simulink model "nonlin_unique_plane"  (Simulink 6.0)
settings: Solver=ode45  StartTime=0.0  StopTime=300  RelTol=1e-3
undefined symbols (not defined in the file): B, DQ, DQL, I, m, M, Ma, MaU, rg, T, W, xb, xg, Xudot, yb, yg, Yvdot, zb, zg, Zwdot
libraries: simulink x24, rov_design_analysis x16
(part 1 of 3)
settings Model: LastModifiedBy=c chin

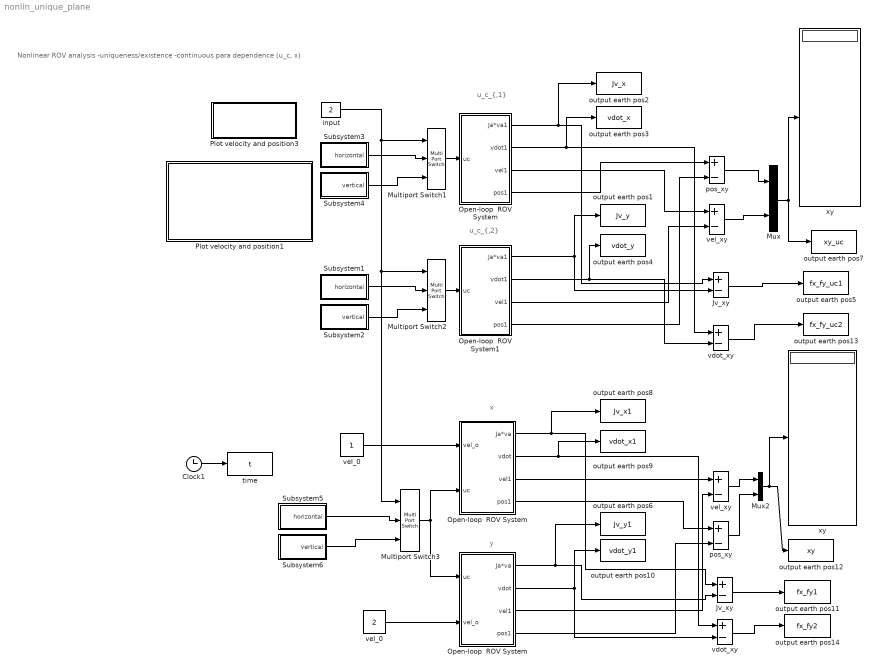
== system nonlin_unique_plane ==
  note: Nonlinear ROV analysis
      | -uniqueness/existence
      | -continuous para dependence (u_c, x)
  note: u_c_{,1}
  note: x
  note: y
  note: u_c_{,2}
  Clock1 : Clock
      settings: Decimation=10
  Jv_xy : Sum  Inputs=+-  SaturateOnIntegerOverflow=on  InputSameDT=on
  "Jv_xy " : Sum  Inputs=+-  SaturateOnIntegerOverflow=on  InputSameDT=on
  Multiport Switch1 : MultiPortSwitch  Inputs=2
  Multiport Switch2 : MultiPortSwitch  Inputs=2
  Multiport Switch3 : MultiPortSwitch  Inputs=2
  Mux : Mux  Inputs=2
  Mux2 : Mux  Inputs=2
  Open-loop  ROV System : Subsystem
  "Open-loop  ROV System   " : Subsystem
  "Open-loop  ROV System     " : Subsystem
  Open-loop  ROV System1 : Subsystem
  Plot velocity and position1 : Subsystem
      settings: OpenFcn=|
      | clc
      | cd C:\Matlab7\toolbox\rov_design_analysis\nonlin_analysis
      | run unique_analy_plane
      mask Display: disp('Double-click \n to \n check \n 1. uniqueness/existence \n 2. continuous  para. dependence\n HORT/VERT')
  Plot velocity and position3 : Subsystem  AncestorBlock=|
      | rov_design_analysis/ROV Controller
      | Design
      | Applications/Plot velocity and position
      settings: OpenFcn=|
      | clc
      | cd c:\Matlab7\toolbox\rov_design_analysis\hybrid
      | sim('nonlin_unique_plane')
      mask Display: disp('Run  SIMULINK')
  Subsystem1 : Subsystem
  Subsystem2 : Subsystem
  Subsystem3 : Subsystem
  Subsystem4 : Subsystem
  Subsystem5 : Subsystem
  Subsystem6 : Subsystem
  "input " : Constant  Value=2
  output earth pos1 : ToWorkspace  VariableName=Jv_y  SampleTime=1  SaveFormat=Array
  output earth pos10 : ToWorkspace  VariableName=vdot_y1  SampleTime=1  SaveFormat=Array
  output earth pos11 : ToWorkspace  VariableName=fx_fy1  SampleTime=1  SaveFormat=Array
  output earth pos12 : ToWorkspace  VariableName=xy  SampleTime=1  SaveFormat=Array
  output earth pos13 : ToWorkspace  VariableName=fx_fy_uc2  SampleTime=1  SaveFormat=Array
  output earth pos14 : ToWorkspace  VariableName=fx_fy2  SampleTime=1  SaveFormat=Array
  output earth pos2 : ToWorkspace  VariableName=Jv_x  SampleTime=1  SaveFormat=Array
  output earth pos3 : ToWorkspace  VariableName=vdot_x  SampleTime=1  SaveFormat=Array
  output earth pos4 : ToWorkspace  VariableName=vdot_y  SampleTime=1  SaveFormat=Array
  output earth pos5 : ToWorkspace  VariableName=fx_fy_uc1  SampleTime=1  SaveFormat=Array
  output earth pos6 : ToWorkspace  VariableName=Jv_y1  SampleTime=1  SaveFormat=Array
  output earth pos7 : ToWorkspace  VariableName=xy_uc  SampleTime=1  SaveFormat=Array
  output earth pos8 : ToWorkspace  VariableName=Jv_x1  SampleTime=1  SaveFormat=Array
  output earth pos9 : ToWorkspace  VariableName=vdot_x1  SampleTime=1  SaveFormat=Array
  pos_xy : Sum  Inputs=+-  SaturateOnIntegerOverflow=on  InputSameDT=on
  "pos_xy " : Sum  Inputs=+-  SaturateOnIntegerOverflow=on  InputSameDT=on
  time : ToWorkspace  VariableName=t  SampleTime=1  SaveFormat=Array
  vdot_xy : Sum  Inputs=+-  SaturateOnIntegerOverflow=on  InputSameDT=on
  "vdot_xy " : Sum  Inputs=+-  SaturateOnIntegerOverflow=on  InputSameDT=on
  vel_0 : Constant  Value=2
  "vel_0 " : Constant
  vel_xy : Sum  Inputs=+-  SaturateOnIntegerOverflow=on  InputSameDT=on
  "vel_xy " : Sum  Inputs=+-  SaturateOnIntegerOverflow=on  InputSameDT=on
  xy : Display
  "xy  " : Display
  wires:
  Clock1/1 -> time/1
  "vel_xy "/1 -> Mux2/1
  "pos_xy "/1 -> Mux2/2
  Mux2/1 -> output earth pos12/1, "xy  "/1
  "vel_0 "/1 -> "Open-loop  ROV System   "/1(vel_o)
  vel_0/1 -> "Open-loop  ROV System     "/2(vel_o)
  Multiport Switch1/1 -> Open-loop  ROV System/1(uc)
  Open-loop  ROV System/1(Ja*va1) -> Jv_xy/1, output earth pos2/1
  Open-loop  ROV System1/1(Ja*va1) -> Jv_xy/2, output earth pos1/1
  Open-loop  ROV System/2(vdot1) -> vdot_xy/1, output earth pos3/1
  Open-loop  ROV System1/2(vdot1) -> vdot_xy/2, output earth pos4/1
  Open-loop  ROV System/4("pos1 ") -> pos_xy/1
  Open-loop  ROV System1/4("pos1 ") -> pos_xy/2
  Open-loop  ROV System/3("vel1 ") -> vel_xy/1
  Open-loop  ROV System1/3("vel1 ") -> vel_xy/2
  pos_xy/1 -> Mux/1
  vel_xy/1 -> Mux/2
  "Open-loop  ROV System   "/1(Ja*va) -> "Jv_xy "/1, output earth pos8/1
  "Open-loop  ROV System     "/1(Ja*va) -> "Jv_xy "/2, output earth pos6/1
  "Open-loop  ROV System   "/3(vel1) -> "vel_xy "/1
  "Open-loop  ROV System     "/3(vel1) -> "vel_xy "/2
  "Open-loop  ROV System   "/4(pos1) -> "pos_xy "/1
  "Open-loop  ROV System     "/4(pos1) -> "pos_xy "/2
  Jv_xy/1 -> output earth pos5/1
  vdot_xy/1 -> output earth pos13/1
  "Jv_xy "/1 -> output earth pos11/1
  "vdot_xy "/1 -> output earth pos14/1
  "Open-loop  ROV System   "/2(vdot) -> "vdot_xy "/1, output earth pos9/1
  "Open-loop  ROV System     "/2(vdot) -> "vdot_xy "/2, output earth pos10/1
  Mux/1 -> output earth pos7/1, xy/1
  Multiport Switch2/1 -> Open-loop  ROV System1/1(uc)
  Multiport Switch3/1 -> "Open-loop  ROV System   "/2(uc), "Open-loop  ROV System     "/1(uc)
  Subsystem4/1(vertical) -> Multiport Switch1/3
  Subsystem3/1(horizontal) -> Multiport Switch1/2
  "input "/1 -> Multiport Switch1/1, Multiport Switch2/1, Multiport Switch3/1
  Subsystem2/1(vertical) -> Multiport Switch2/3
  Subsystem1/1(horizontal) -> Multiport Switch2/2
  Subsystem6/1(vertical) -> Multiport Switch3/3
  Subsystem5/1(horizontal) -> Multiport Switch3/2

== system nonlin_unique_plane/Open-loop  ROV System ==
  uc : Inport  Port=1  LatchInput=off
  " Six DOF RRC ROV   " : Subsystem
      mask Display:
      | disp('ROV')
      | image(imread('/rov_design_analysis/fig/ROVRRC2.jpg'));
      | color('white');port_label('input',2,'thrust')
      | color('white');port_label('input',1,'MCD_select')
      | color('white');port_label('input',3,'pos')
      | color('white');port_label('output',1,'vel')
      | color('white');port_label('output',2,'vel_dot')
  Body Velocity Scope  1 : Subsystem  AncestorBlock=|
      | rov_design_analysis/Scope
      | Utilities/Body Velocity
      | Scope
      mask Display: disp('Body\nVelocity\nScope')
  "Euler Transformation  " : Subsystem  AncestorBlock=rov_design_analysis/Scope Utilities/Euler Transformation
  Thruster configuration5 : Subsystem
      mask Display: disp('T')
  Thruster configuration8 : Subsystem  AncestorBlock=|
      | rov_design_analysis/ROV Controller
      | Design
      | Applications/1. Heading autopilot/Thruster
      | configuration
      mask Display: disp('F_T')
  "input " : Constant  Value=2
  Ja*va1 : Outport
  vdot1 : Outport  Port=2
  "vel1 " : Outport  Port=3
  "pos1 " : Outport  Port=4
  wires:
  "Euler Transformation  "/1(eout) -> Body Velocity Scope  1/1(In), "pos1 "/1, " Six DOF RRC ROV   "/3("pos ")
  " Six DOF RRC ROV   "/1(vel) -> "Euler Transformation  "/1(vel), "vel1 "/1
  " Six DOF RRC ROV   "/2(vel_dot) -> vdot1/1
  "Euler Transformation  "/2(eout_dot) -> Ja*va1/1
  Thruster configuration8/1(output force) -> Thruster configuration5/1(input velocity)
  Thruster configuration5/1(output force) -> " Six DOF RRC ROV   "/2("thrust ")
  uc/1 -> Thruster configuration8/1(input velocity)
  "input "/1 -> " Six DOF RRC ROV   "/1(MCD_select)

== system nonlin_unique_plane/Open-loop  ROV System    ==
  vel_o : Inport  Port=1  LatchInput=off
  uc : Inport  Port=2  LatchInput=off
  " Six DOF RRC ROV   " : Subsystem
      mask Display:
      | disp('ROV')
      | image(imread('/rov_design_analysis/fig/ROVRRC2.jpg'));
      | color('white');port_label('input',2,'thrust')
      | color('white');port_label('input',1,'MCD_select')
      | color('white');port_label('input',3,'pos')
      | color('white');port_label('output',1,'vel')
      | color('white');port_label('output',2,'vel_dot')
  Body Velocity Scope  1 : Subsystem  AncestorBlock=|
      | rov_design_analysis/Scope
      | Utilities/Body Velocity
      | Scope
      mask Display: disp('Body\nVelocity\nScope')
  "Euler Transformation  " : Subsystem  AncestorBlock=rov_design_analysis/Scope Utilities/Euler Transformation
  Thruster configuration5 : Subsystem
      mask Display: disp('T')
  Thruster configuration8 : Subsystem  AncestorBlock=|
      | rov_design_analysis/ROV Controller
      | Design
      | Applications/1. Heading autopilot/Thruster
      | configuration
      mask Display: disp('F_T')
  "input " : Constant  Value=2
  Ja*va : Outport
  vdot : Outport  Port=2
  vel1 : Outport  Port=3
  pos1 : Outport  Port=4
  wires:
  "Euler Transformation  "/1(eout) -> pos1/1, " Six DOF RRC ROV   "/3("pos "), Body Velocity Scope  1/1(In)
  " Six DOF RRC ROV   "/1(vel) -> "Euler Transformation  "/1(vel), vel1/1
  "Euler Transformation  "/2(Ja*va) -> Ja*va/1
  " Six DOF RRC ROV   "/2(vel_dot) -> vdot/1
  vel_o/1 -> " Six DOF RRC ROV   "/4(v0)
  Thruster configuration8/1(output force) -> Thruster configuration5/1(input velocity)
  Thruster configuration5/1(output force) -> " Six DOF RRC ROV   "/2("thrust ")
  uc/1 -> Thruster configuration8/1(input velocity)
  "input "/1 -> " Six DOF RRC ROV   "/1(MCD_select)

== system nonlin_unique_plane/Open-loop  ROV System      ==
  uc : Inport  Port=1  LatchInput=off
  vel_o : Inport  Port=2  LatchInput=off
  " Six DOF RRC ROV   " : Subsystem
      mask Display:
      | disp('ROV')
      | image(imread('/rov_design_analysis/fig/ROVRRC2.jpg'));
      | color('white');port_label('input',2,'thrust')
      | color('white');port_label('input',1,'MCD_select')
      | color('white');port_label('input',3,'pos')
      | color('white');port_label('output',1,'vel')
      | color('white');port_label('output',2,'vel_dot')
  Body Velocity Scope  1 : Subsystem  AncestorBlock=|
      | rov_design_analysis/Scope
      | Utilities/Body Velocity
      | Scope
      mask Display: disp('Body\nVelocity\nScope')
  "Euler Transformation  " : Subsystem  AncestorBlock=rov_design_analysis/Scope Utilities/Euler Transformation
  Thruster configuration5 : Subsystem
      mask Display: disp('T')
  Thruster configuration8 : Subsystem  AncestorBlock=|
      | rov_design_analysis/ROV Controller
      | Design
      | Applications/1. Heading autopilot/Thruster
      | configuration
      mask Display: disp('F_T')
  "input " : Constant  Value=2
  Ja*va : Outport
  vdot : Outport  Port=2
  vel1 : Outport  Port=3
  pos1 : Outport  Port=4
  wires:
  "Euler Transformation  "/1(eout) -> pos1/1, " Six DOF RRC ROV   "/3("pos "), Body Velocity Scope  1/1(In)
  " Six DOF RRC ROV   "/1(vel) -> "Euler Transformation  "/1(vel), vel1/1
  "Euler Transformation  "/2(Ja*va) -> Ja*va/1
  " Six DOF RRC ROV   "/2(vel_dot) -> vdot/1
  vel_o/1 -> " Six DOF RRC ROV   "/4(v0)
  Thruster configuration8/1(output force) -> Thruster configuration5/1(input velocity)
  Thruster configuration5/1(output force) -> " Six DOF RRC ROV   "/2("thrust ")
  uc/1 -> Thruster configuration8/1(input velocity)
  "input "/1 -> " Six DOF RRC ROV   "/1(MCD_select)

== system nonlin_unique_plane/Open-loop  ROV System1 ==
  uc : Inport  Port=1  LatchInput=off
  " Six DOF RRC ROV   " : Subsystem
      mask Display:
      | disp('ROV')
      | image(imread('/rov_design_analysis/fig/ROVRRC2.jpg'));
      | color('white');port_label('input',2,'thrust')
      | color('white');port_label('input',1,'MCD_select')
      | color('white');port_label('input',3,'pos')
      | color('white');port_label('output',1,'vel')
      | color('white');port_label('output',2,'vel_dot')
  Body Velocity Scope  1 : Subsystem  AncestorBlock=|
      | rov_design_analysis/Scope
      | Utilities/Body Velocity
      | Scope
      mask Display: disp('Body\nVelocity\nScope')
  "Euler Transformation  " : Subsystem  AncestorBlock=rov_design_analysis/Scope Utilities/Euler Transformation
  Thruster configuration5 : Subsystem
      mask Display: disp('T')
  Thruster configuration8 : Subsystem  AncestorBlock=|
      | rov_design_analysis/ROV Controller
      | Design
      | Applications/1. Heading autopilot/Thruster
      | configuration
      mask Display: disp('F_T')
  "input " : Constant  Value=2
  Ja*va1 : Outport
  vdot1 : Outport  Port=2
  "vel1 " : Outport  Port=3
  "pos1 " : Outport  Port=4
  wires:
  "Euler Transformation  "/1(eout) -> "pos1 "/1, Body Velocity Scope  1/1(In), " Six DOF RRC ROV   "/3("pos ")
  " Six DOF RRC ROV   "/1(vel) -> "Euler Transformation  "/1(vel), "vel1 "/1
  " Six DOF RRC ROV   "/2(vel_dot) -> vdot1/1
  "Euler Transformation  "/2(eout_dot) -> Ja*va1/1
  Thruster configuration8/1(output force) -> Thruster configuration5/1(input velocity)
  Thruster configuration5/1(output force) -> " Six DOF RRC ROV   "/2("thrust ")
  uc/1 -> Thruster configuration8/1(input velocity)
  "input "/1 -> " Six DOF RRC ROV   "/1(MCD_select)

== system nonlin_unique_plane/Plot velocity and position1 ==

== system nonlin_unique_plane/Plot velocity and position3 ==

== system nonlin_unique_plane/Subsystem1 ==
  Mux1 : Mux
  u1 : Step  Time=0  After=2  SampleTime=0
  u2 : Step  Time=0  After=2  SampleTime=0
  u3 : Step  Time=0  After=0  SampleTime=0
  u4 : Step  Time=0  After=0  SampleTime=0
  horizontal : Outport
  wires:
  u2/1 -> Mux1/2
  u1/1 -> Mux1/1
  u3/1 -> Mux1/3
  Mux1/1 -> horizontal/1
  u4/1 -> Mux1/4

== system nonlin_unique_plane/Subsystem2 ==
  Mux1 : Mux
  u1 : Step  Time=0  After=0  SampleTime=0
  u2 : Step  Time=0  After=0  SampleTime=0
  u3 : Step  Time=0  After=2  SampleTime=0
  u4 : Step  Time=0  After=2  SampleTime=0
  vertical : Outport
  wires:
  u2/1 -> Mux1/2
  u1/1 -> Mux1/1
  u3/1 -> Mux1/3
  u4/1 -> Mux1/4
  Mux1/1 -> vertical/1

== system nonlin_unique_plane/Subsystem3 ==
  Mux1 : Mux
  u1 : Step  Time=0  SampleTime=0
  u2 : Step  Time=0  SampleTime=0
  u3 : Step  Time=0  After=0  SampleTime=0
  u4 : Step  Time=0  After=0  SampleTime=0
  horizontal : Outport
  wires:
  u2/1 -> Mux1/2
  u1/1 -> Mux1/1
  u3/1 -> Mux1/3
  Mux1/1 -> horizontal/1
  u4/1 -> Mux1/4

== system nonlin_unique_plane/Subsystem4 ==
  Mux1 : Mux
  u1 : Step  Time=0  After=0  SampleTime=0
  u2 : Step  Time=0  After=0  SampleTime=0
  u3 : Step  Time=0  SampleTime=0
  u4 : Step  Time=0  SampleTime=0
  vertical : Outport
  wires:
  u2/1 -> Mux1/2
  u1/1 -> Mux1/1
  u3/1 -> Mux1/3
  u4/1 -> Mux1/4
  Mux1/1 -> vertical/1

== system nonlin_unique_plane/Subsystem5 ==
  Mux1 : Mux
  u1 : Step  Time=0  SampleTime=0
  u2 : Step  Time=0  SampleTime=0
  u3 : Step  Time=0  After=0  SampleTime=0
  u4 : Step  Time=0  After=0  SampleTime=0
  horizontal : Outport
  wires:
  u2/1 -> Mux1/2
  u1/1 -> Mux1/1
  u3/1 -> Mux1/3
  Mux1/1 -> horizontal/1
  u4/1 -> Mux1/4

== system nonlin_unique_plane/Subsystem6 ==
  Mux1 : Mux
  u1 : Step  Time=0  After=0  SampleTime=0
  u2 : Step  Time=0  After=0  SampleTime=0
  u3 : Step  Time=0  SampleTime=0
  u4 : Step  Time=0  SampleTime=0
  vertical : Outport
  wires:
  u2/1 -> Mux1/2
  u1/1 -> Mux1/1
  u3/1 -> Mux1/3
  u4/1 -> Mux1/4
  Mux1/1 -> vertical/1

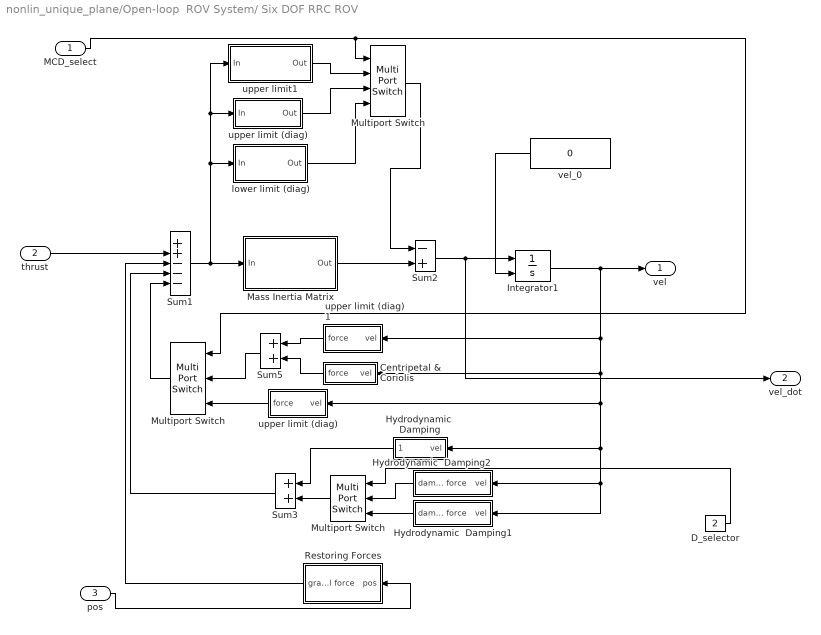
== system nonlin_unique_plane/Open-loop  ROV System/ Six DOF RRC ROV    ==
  MCD_select : Inport  Port=1  LatchInput=off
  "thrust " : Inport  Port=2  LatchInput=off
  "pos " : Inport  Port=3  LatchInput=off
  Centripetal & Coriolis : Subsystem  Orientation=left  AncestorBlock=rov_design_analysis/ROV Models/1. Six DOF RRC ROV II/Centripetal & Coriolis
      mask Display: disp('C')
  D_selector : Constant  Value=2
  Hydrodynamic  Damping : Subsystem  Orientation=left
      mask Display: disp('D')
  Hydrodynamic  Damping1 : Subsystem  Orientation=left
      mask Display: disp('perturb \nDamping')
  Hydrodynamic  Damping2 : Subsystem  Orientation=left
      mask Display: disp('Zero Perturb')
  Integrator1 : Integrator  InitialConditionSource=external
  Mass Inertia Matrix : Subsystem
      mask Display: disp('inv(MRB+MA)')
  Multiport Switch : MultiPortSwitch  Inputs=3
  "Multiport Switch  " : MultiPortSwitch  Orientation=left  Inputs=2
  "Multiport Switch    " : MultiPortSwitch  Orientation=left  Inputs=2
  Restoring Forces : Subsystem  Orientation=left
      mask Display: disp('Restoring\nForce')
  Sum1 : Sum  Inputs=++---  SaturateOnIntegerOverflow=on  InputSameDT=on
  Sum2 : Sum  Inputs=-+  SaturateOnIntegerOverflow=on  InputSameDT=on
  Sum3 : Sum  Orientation=left  SaturateOnIntegerOverflow=on  InputSameDT=on
  Sum5 : Sum  Orientation=left  SaturateOnIntegerOverflow=on  InputSameDT=on
  lower limit (diag) : Subsystem
      mask Display: disp('Perturb MA')
  upper limit (diag) : Subsystem
      mask Display: disp('Perturb MA')
  "upper limit (diag)   " : Subsystem  Orientation=left
      mask Display: disp('Perturb CA')
  upper limit (diag)   1 : Subsystem  Orientation=left
      mask Display: disp('CA')
  upper limit1 : Subsystem
      mask Display: disp('Zero Perturb')
  vel_0 : Constant  Orientation=left  Value=0  OutDataTypeMode=double
  vel : Outport
  vel_dot : Outport  Port=2
  wires:
  Restoring Forces/1(gravitational force) -> Sum1/3
  "thrust "/1 -> Sum1/2
  Sum1/1 -> Mass Inertia Matrix/1(In), upper limit1/1(In), upper limit (diag)/1(In), lower limit (diag)/1(In)
  "Multiport Switch  "/1 -> Sum1/5
  "pos "/1 -> Restoring Forces/1(pos)
  Mass Inertia Matrix/1(Out) -> Sum2/2
  upper limit1/1(Out) -> Multiport Switch/2
  upper limit (diag)/1(Out) -> Multiport Switch/3
  lower limit (diag)/1(Out) -> Multiport Switch/4
  Multiport Switch/1 -> Sum2/1
  "upper limit (diag)   "/1(force) -> "Multiport Switch  "/3
  Sum5/1 -> "Multiport Switch  "/2
  Hydrodynamic  Damping1/1(damping force) -> "Multiport Switch    "/3
  Hydrodynamic  Damping2/1(damping force) -> "Multiport Switch    "/2
  Sum3/1 -> Sum1/4
  "Multiport Switch    "/1 -> Sum3/2
  Hydrodynamic  Damping/1(damping force) -> Sum3/1
  MCD_select/1 -> Multiport Switch/1, "Multiport Switch  "/1
  upper limit (diag)   1/1(force) -> Sum5/1
  Centripetal & Coriolis/1(force) -> Sum5/2
  Sum2/1 -> Integrator1/1, vel_dot/1
  Integrator1/1 -> vel/1, upper limit (diag)   1/1(vel), Centripetal & Coriolis/1(vel), Hydrodynamic  Damping/1(vel), Hydrodynamic  Damping1/1(vel), Hydrodynamic  Damping2/1(vel), "upper limit (diag)   "/1(vel)
  vel_0/1 -> Integrator1/2
  D_selector/1 -> "Multiport Switch    "/1

== system nonlin_unique_plane/Open-loop  ROV System/Body Velocity Scope  1 ==
  In : Inport  Port=1  LatchInput=off
  Demux : Demux  Outputs=6
  p : Scope
      settings: TickLabels=on  YMin=-0.125  YMax=0.2  DataFormat=Array
  q : Scope
      settings: TickLabels=on  TimeRange=200  YMin=-0.05  YMax=0.15  DataFormat=Array
  r : Scope
      settings: TickLabels=on  TimeRange=200  YMin=-0.05  YMax=0.15  DataFormat=Array
  u : Scope
      settings: TickLabels=on  TimeRange=50  YMin=-0.025  YMax=0.375  DataFormat=Array
  v : Scope
      settings: TickLabels=on  YMin=-0.02  YMax=0.1  DataFormat=Array
  w : Scope
      settings: TickLabels=on  TimeRange=50  YMin=-0.0025  YMax=0.0375  DataFormat=Array
  wires:
  Demux/1 -> u/1
  Demux/2 -> v/1
  Demux/4 -> p/1
  Demux/3 -> w/1
  In/1 -> Demux/1
  Demux/5 -> q/1
  Demux/6 -> r/1

== system nonlin_unique_plane/Open-loop  ROV System/Euler Transformation   ==
  vel : Inport  Port=1  LatchInput=off
  Demux : Demux  Outputs=2
  Demux1 : Demux  Outputs=2
  Intregrator2 : Integrator
  Mux1 : Mux  Inputs=2
  Terminator : Terminator
  Transformation matrix R : Subsystem
      mask Display: disp('Transformation R')
  Transformation matrix T : Subsystem
      mask Display: disp('Transformation T')
  eout : Outport  InitialOutput=0
  eout_dot : Outport  Port=2  InitialOutput=0
  wires:
  Mux1/1 -> eout_dot/1, Intregrator2/1
  Intregrator2/1 -> Demux1/1, eout/1
  Demux/2 -> Transformation matrix R/1(angular body  velocity)
  Demux/1 -> Transformation matrix T/1(translational body velocity)
  vel/1 -> Demux/1
  Demux1/2 -> Transformation matrix T/2(angular position), Transformation matrix R/2(angular position)
  Transformation matrix R/1(angular earth velocity) -> Mux1/2
  Transformation matrix T/1(translational earth velocity) -> Mux1/1
  Demux1/1 -> Terminator/1

== system nonlin_unique_plane/Open-loop  ROV System/Thruster configuration5 ==
  input velocity : Inport  Orientation=up  Port=1  LatchInput=off
  Thruster Matrix : Gain  Gain=T  Multiplication=Matrix(K*u)  SaturateOnIntegerOverflow=on
  output force : Outport  InitialOutput=0
  wires:
  input velocity/1 -> Thruster Matrix/1
  Thruster Matrix/1 -> output force/1

== system nonlin_unique_plane/Open-loop  ROV System/Thruster configuration8 ==
  input velocity : Inport  Orientation=up  Port=1  LatchInput=off
  3. propeller with motor characteristics - 1DoF (no account for ua,up){,1..3} (4 alike) : rov_design_analysis/Propeller Models/3. propeller with motor characteristics - 1DoF (no account for ua,up)
  Demux : Demux
  Mux1 : Mux
  output force : Outport  InitialOutput=0
  wires:
  3. propeller with motor characteristics - 1DoF (no account for ua,up)/1 -> Mux1/1
  3. propeller with motor characteristics - 1DoF (no account for ua,up)1/1 -> Mux1/2
  3. propeller with motor characteristics - 1DoF (no account for ua,up)2/1 -> Mux1/3
  3. propeller with motor characteristics - 1DoF (no account for ua,up)3/1 -> Mux1/4
  Mux1/1 -> output force/1
  input velocity/1 -> Demux/1
  Demux/1 -> 3. propeller with motor characteristics - 1DoF (no account for ua,up)/1
  Demux/2 -> 3. propeller with motor characteristics - 1DoF (no account for ua,up)1/1
  Demux/3 -> 3. propeller with motor characteristics - 1DoF (no account for ua,up)2/1
  Demux/4 -> 3. propeller with motor characteristics - 1DoF (no account for ua,up)3/1

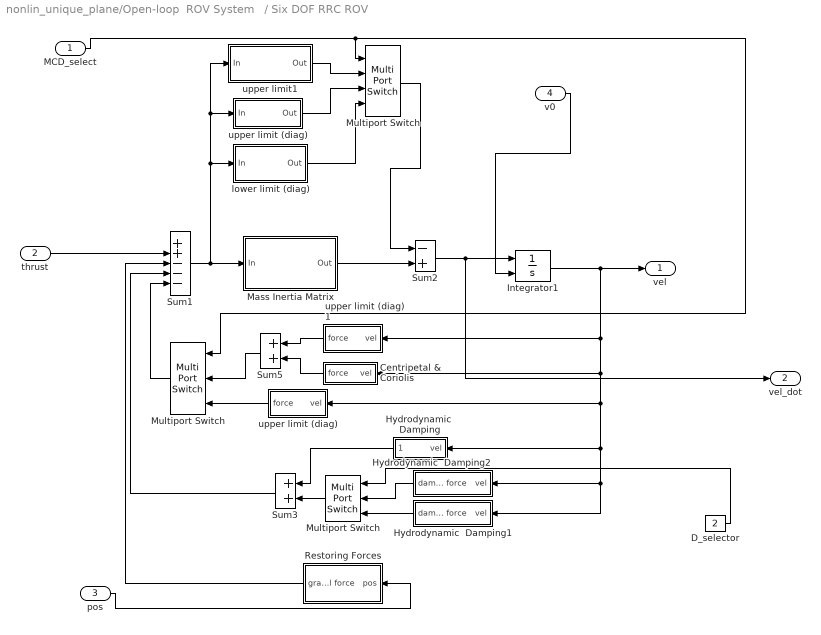
== system nonlin_unique_plane/Open-loop  ROV System   / Six DOF RRC ROV    ==
  MCD_select : Inport  Port=1  LatchInput=off
  "thrust " : Inport  Port=2  LatchInput=off
  "pos " : Inport  Port=3  LatchInput=off
  v0 : Inport  Port=4  LatchInput=off
  Centripetal & Coriolis : Subsystem  Orientation=left  AncestorBlock=rov_design_analysis/ROV Models/1. Six DOF RRC ROV II/Centripetal & Coriolis
      mask Display: disp('C')
  D_selector : Constant  Value=2
  Hydrodynamic  Damping : Subsystem  Orientation=left
      mask Display: disp('D')
  Hydrodynamic  Damping1 : Subsystem  Orientation=left
      mask Display: disp('perturb \nDamping')
  Hydrodynamic  Damping2 : Subsystem  Orientation=left
      mask Display: disp('Zero Perturb')
  Integrator1 : Integrator  InitialConditionSource=external
  Mass Inertia Matrix : Subsystem
      mask Display: disp('inv(MRB+MA)')
  Multiport Switch : MultiPortSwitch  Inputs=3
  "Multiport Switch  " : MultiPortSwitch  Orientation=left  Inputs=2
  "Multiport Switch    " : MultiPortSwitch  Orientation=left  Inputs=2
  Restoring Forces : Subsystem  Orientation=left
      mask Display: disp('Restoring\nForce')
  Sum1 : Sum  Inputs=++---  SaturateOnIntegerOverflow=on  InputSameDT=on
  Sum2 : Sum  Inputs=-+  SaturateOnIntegerOverflow=on  InputSameDT=on
  Sum3 : Sum  Orientation=left  SaturateOnIntegerOverflow=on  InputSameDT=on
  Sum5 : Sum  Orientation=left  SaturateOnIntegerOverflow=on  InputSameDT=on
  lower limit (diag) : Subsystem
      mask Display: disp('Perturb MA')
  upper limit (diag) : Subsystem
      mask Display: disp('Perturb MA')
  "upper limit (diag)   " : Subsystem  Orientation=left
      mask Display: disp('Perturb CA')
  upper limit (diag)   1 : Subsystem  Orientation=left
      mask Display: disp('CA')
  upper limit1 : Subsystem
      mask Display: disp('Zero Perturb')
  vel : Outport
  vel_dot : Outport  Port=2
  wires:
  Restoring Forces/1(gravitational force) -> Sum1/3
  "thrust "/1 -> Sum1/2
  Sum1/1 -> Mass Inertia Matrix/1(In), upper limit1/1(In), upper limit (diag)/1(In), lower limit (diag)/1(In)
  "Multiport Switch  "/1 -> Sum1/5
  "pos "/1 -> Restoring Forces/1(pos)
  Mass Inertia Matrix/1(Out) -> Sum2/2
  upper limit1/1(Out) -> Multiport Switch/2
  upper limit (diag)/1(Out) -> Multiport Switch/3
  lower limit (diag)/1(Out) -> Multiport Switch/4
  Multiport Switch/1 -> Sum2/1
  "upper limit (diag)   "/1(force) -> "Multiport Switch  "/3
  Sum5/1 -> "Multiport Switch  "/2
  Hydrodynamic  Damping1/1(damping force) -> "Multiport Switch    "/3
  Hydrodynamic  Damping2/1(damping force) -> "Multiport Switch    "/2
  Sum3/1 -> Sum1/4
  "Multiport Switch    "/1 -> Sum3/2
  Hydrodynamic  Damping/1(damping force) -> Sum3/1
  MCD_select/1 -> "Multiport Switch  "/1, Multiport Switch/1
  upper limit (diag)   1/1(force) -> Sum5/1
  Centripetal & Coriolis/1(force) -> Sum5/2
  Sum2/1 -> Integrator1/1, vel_dot/1
  Integrator1/1 -> vel/1, upper limit (diag)   1/1(vel), Centripetal & Coriolis/1(vel), Hydrodynamic  Damping/1(vel), Hydrodynamic  Damping1/1(vel), Hydrodynamic  Damping2/1(vel), "upper limit (diag)   "/1(vel)
  v0/1 -> Integrator1/2
  D_selector/1 -> "Multiport Switch    "/1

== system nonlin_unique_plane/Open-loop  ROV System   /Body Velocity Scope  1 ==
  In : Inport  Port=1  LatchInput=off
  Demux : Demux  Outputs=6
  p : Scope
      settings: TickLabels=on  YMin=-0.125  YMax=0.2  DataFormat=Array
  q : Scope
      settings: TickLabels=on  TimeRange=200  YMin=-0.05  YMax=0.15  DataFormat=Array
  r : Scope
      settings: TickLabels=on  TimeRange=200  YMin=-0.05  YMax=0.15  DataFormat=Array
  u : Scope
      settings: TickLabels=on  TimeRange=50  YMin=-0.025  YMax=0.375  DataFormat=Array
  v : Scope
      settings: TickLabels=on  YMin=-0.02  YMax=0.1  DataFormat=Array
  w : Scope
      settings: TickLabels=on  TimeRange=50  YMin=-0.0025  YMax=0.0375  DataFormat=Array
  wires:
  Demux/1 -> u/1
  Demux/2 -> v/1
  Demux/4 -> p/1
  Demux/3 -> w/1
  In/1 -> Demux/1
  Demux/5 -> q/1
  Demux/6 -> r/1

== system nonlin_unique_plane/Open-loop  ROV System   /Euler Transformation   ==
  vel : Inport  Port=1  LatchInput=off
  Demux : Demux  Outputs=2
  Demux1 : Demux  Outputs=2
  Intregrator2 : Integrator
  Mux1 : Mux  Inputs=2
  Terminator : Terminator
  Transformation matrix R : Subsystem
      mask Display: disp('Transformation R')
  Transformation matrix T : Subsystem
      mask Display: disp('Transformation T')
  eout : Outport  InitialOutput=0
  Ja*va : Outport  Port=2  InitialOutput=0
  wires:
  Mux1/1 -> Ja*va/1, Intregrator2/1
  Intregrator2/1 -> Demux1/1, eout/1
  Demux/2 -> Transformation matrix R/1(angular body  velocity)
  Demux/1 -> Transformation matrix T/1(translational body velocity)
  vel/1 -> Demux/1
  Demux1/2 -> Transformation matrix T/2(angular position), Transformation matrix R/2(angular position)
  Transformation matrix R/1(angular earth velocity) -> Mux1/2
  Transformation matrix T/1(translational earth velocity) -> Mux1/1
  Demux1/1 -> Terminator/1

== system nonlin_unique_plane/Open-loop  ROV System   /Thruster configuration5 ==
  input velocity : Inport  Orientation=up  Port=1  LatchInput=off
  Thruster Matrix : Gain  Gain=T  Multiplication=Matrix(K*u)  SaturateOnIntegerOverflow=on
  output force : Outport  InitialOutput=0
  wires:
  input velocity/1 -> Thruster Matrix/1
  Thruster Matrix/1 -> output force/1

== system nonlin_unique_plane/Open-loop  ROV System   /Thruster configuration8 ==
  input velocity : Inport  Orientation=up  Port=1  LatchInput=off
  3. propeller with motor characteristics - 1DoF (no account for ua,up){,1..3} (4 alike) : rov_design_analysis/Propeller Models/3. propeller with motor characteristics - 1DoF (no account for ua,up)
  Demux : Demux
  Mux1 : Mux
  output force : Outport  InitialOutput=0
  wires:
  3. propeller with motor characteristics - 1DoF (no account for ua,up)/1 -> Mux1/1
  3. propeller with motor characteristics - 1DoF (no account for ua,up)1/1 -> Mux1/2
  3. propeller with motor characteristics - 1DoF (no account for ua,up)2/1 -> Mux1/3
  3. propeller with motor characteristics - 1DoF (no account for ua,up)3/1 -> Mux1/4
  Mux1/1 -> output force/1
  input velocity/1 -> Demux/1
  Demux/1 -> 3. propeller with motor characteristics - 1DoF (no account for ua,up)/1
  Demux/2 -> 3. propeller with motor characteristics - 1DoF (no account for ua,up)1/1
  Demux/3 -> 3. propeller with motor characteristics - 1DoF (no account for ua,up)2/1
  Demux/4 -> 3. propeller with motor characteristics - 1DoF (no account for ua,up)3/1

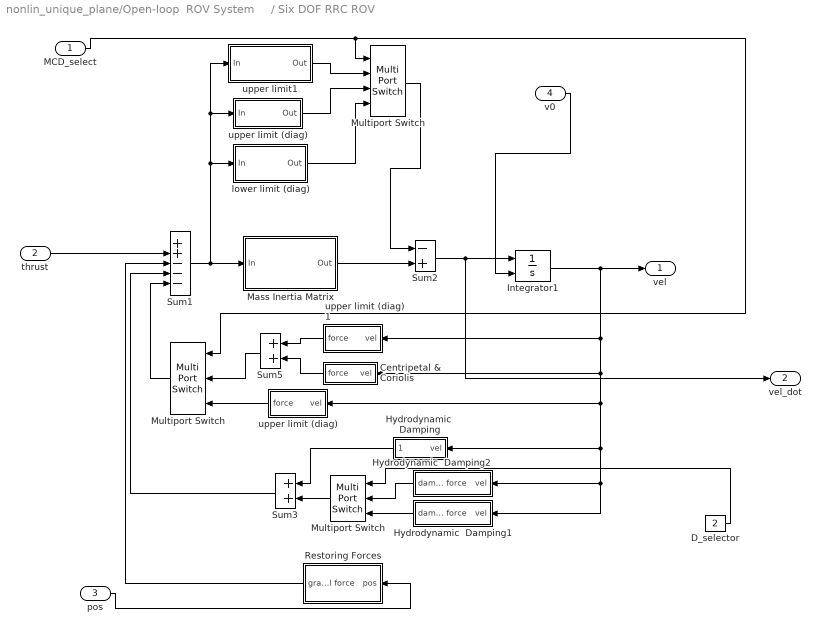
== system nonlin_unique_plane/Open-loop  ROV System     / Six DOF RRC ROV    ==
  MCD_select : Inport  Port=1  LatchInput=off
  "thrust " : Inport  Port=2  LatchInput=off
  "pos " : Inport  Port=3  LatchInput=off
  v0 : Inport  Port=4  LatchInput=off
  Centripetal & Coriolis : Subsystem  Orientation=left  AncestorBlock=rov_design_analysis/ROV Models/1. Six DOF RRC ROV II/Centripetal & Coriolis
      mask Display: disp('C')
  D_selector : Constant  Value=2
  Hydrodynamic  Damping : Subsystem  Orientation=left
      mask Display: disp('D')
  Hydrodynamic  Damping1 : Subsystem  Orientation=left
      mask Display: disp('perturb \nDamping')
  Hydrodynamic  Damping2 : Subsystem  Orientation=left
      mask Display: disp('Zero Perturb')
  Integrator1 : Integrator  InitialConditionSource=external
  Mass Inertia Matrix : Subsystem
      mask Display: disp('inv(MRB+MA)')
  Multiport Switch : MultiPortSwitch  Inputs=3
  "Multiport Switch  " : MultiPortSwitch  Orientation=left  Inputs=2
  "Multiport Switch    " : MultiPortSwitch  Orientation=left  Inputs=2
  Restoring Forces : Subsystem  Orientation=left
      mask Display: disp('Restoring\nForce')
  Sum1 : Sum  Inputs=++---  SaturateOnIntegerOverflow=on  InputSameDT=on
  Sum2 : Sum  Inputs=-+  SaturateOnIntegerOverflow=on  InputSameDT=on
  Sum3 : Sum  Orientation=left  SaturateOnIntegerOverflow=on  InputSameDT=on
  Sum5 : Sum  Orientation=left  SaturateOnIntegerOverflow=on  InputSameDT=on
  lower limit (diag) : Subsystem
      mask Display: disp('Perturb MA')
  upper limit (diag) : Subsystem
      mask Display: disp('Perturb MA')
  "upper limit (diag)   " : Subsystem  Orientation=left
      mask Display: disp('Perturb CA')
  upper limit (diag)   1 : Subsystem  Orientation=left
      mask Display: disp('CA')
  upper limit1 : Subsystem
      mask Display: disp('Zero Perturb')
  vel : Outport
  vel_dot : Outport  Port=2
  wires:
  Restoring Forces/1(gravitational force) -> Sum1/3
  "thrust "/1 -> Sum1/2
  Sum1/1 -> Mass Inertia Matrix/1(In), upper limit1/1(In), upper limit (diag)/1(In), lower limit (diag)/1(In)
  "Multiport Switch  "/1 -> Sum1/5
  "pos "/1 -> Restoring Forces/1(pos)
  Mass Inertia Matrix/1(Out) -> Sum2/2
  upper limit1/1(Out) -> Multiport Switch/2
  upper limit (diag)/1(Out) -> Multiport Switch/3
  lower limit (diag)/1(Out) -> Multiport Switch/4
  Multiport Switch/1 -> Sum2/1
  "upper limit (diag)   "/1(force) -> "Multiport Switch  "/3
  Sum5/1 -> "Multiport Switch  "/2
  Hydrodynamic  Damping1/1(damping force) -> "Multiport Switch    "/3
  Hydrodynamic  Damping2/1(damping force) -> "Multiport Switch    "/2
  Sum3/1 -> Sum1/4
  "Multiport Switch    "/1 -> Sum3/2
  Hydrodynamic  Damping/1(damping force) -> Sum3/1
  MCD_select/1 -> Multiport Switch/1, "Multiport Switch  "/1
  upper limit (diag)   1/1(force) -> Sum5/1
  Centripetal & Coriolis/1(force) -> Sum5/2
  Sum2/1 -> Integrator1/1, vel_dot/1
  Integrator1/1 -> vel/1, upper limit (diag)   1/1(vel), Centripetal & Coriolis/1(vel), Hydrodynamic  Damping/1(vel), Hydrodynamic  Damping1/1(vel), Hydrodynamic  Damping2/1(vel), "upper limit (diag)   "/1(vel)
  v0/1 -> Integrator1/2
  D_selector/1 -> "Multiport Switch    "/1

== system nonlin_unique_plane/Open-loop  ROV System     /Body Velocity Scope  1 ==
  In : Inport  Port=1  LatchInput=off
  Demux : Demux  Outputs=6
  p : Scope
      settings: TickLabels=on  YMin=-0.125  YMax=0.2  DataFormat=Array
  q : Scope
      settings: TickLabels=on  TimeRange=200  YMin=-0.05  YMax=0.15  DataFormat=Array
  r : Scope
      settings: TickLabels=on  TimeRange=200  YMin=-0.05  YMax=0.15  DataFormat=Array
  u : Scope
      settings: TickLabels=on  TimeRange=50  YMin=-0.025  YMax=0.375  DataFormat=Array
  v : Scope
      settings: TickLabels=on  YMin=-0.02  YMax=0.1  DataFormat=Array
  w : Scope
      settings: TickLabels=on  TimeRange=50  YMin=-0.0025  YMax=0.0375  DataFormat=Array
  wires:
  Demux/1 -> u/1
  Demux/2 -> v/1
  Demux/4 -> p/1
  Demux/3 -> w/1
  In/1 -> Demux/1
  Demux/5 -> q/1
  Demux/6 -> r/1

== system nonlin_unique_plane/Open-loop  ROV System     /Euler Transformation   ==
  vel : Inport  Port=1  LatchInput=off
  Demux : Demux  Outputs=2
  Demux1 : Demux  Outputs=2
  Intregrator2 : Integrator
  Mux1 : Mux  Inputs=2
  Terminator : Terminator
  Transformation matrix R : Subsystem
      mask Display: disp('Transformation R')
  Transformation matrix T : Subsystem
      mask Display: disp('Transformation T')
  eout : Outport  InitialOutput=0
  Ja*va : Outport  Port=2  InitialOutput=0
  wires:
  Mux1/1 -> Ja*va/1, Intregrator2/1
  Intregrator2/1 -> Demux1/1, eout/1
  Demux/2 -> Transformation matrix R/1(angular body  velocity)
  Demux/1 -> Transformation matrix T/1(translational body velocity)
  vel/1 -> Demux/1
  Demux1/2 -> Transformation matrix T/2(angular position), Transformation matrix R/2(angular position)
  Transformation matrix R/1(angular earth velocity) -> Mux1/2
  Transformation matrix T/1(translational earth velocity) -> Mux1/1
  Demux1/1 -> Terminator/1

== system nonlin_unique_plane/Open-loop  ROV System     /Thruster configuration5 ==
  input velocity : Inport  Orientation=up  Port=1  LatchInput=off
  Thruster Matrix : Gain  Gain=T  Multiplication=Matrix(K*u)  SaturateOnIntegerOverflow=on
  output force : Outport  InitialOutput=0
  wires:
  input velocity/1 -> Thruster Matrix/1
  Thruster Matrix/1 -> output force/1

== system nonlin_unique_plane/Open-loop  ROV System     /Thruster configuration8 ==
  input velocity : Inport  Orientation=up  Port=1  LatchInput=off
  3. propeller with motor characteristics - 1DoF (no account for ua,up){,1..3} (4 alike) : rov_design_analysis/Propeller Models/3. propeller with motor characteristics - 1DoF (no account for ua,up)
  Demux : Demux
  Mux1 : Mux
  output force : Outport  InitialOutput=0
  wires:
  3. propeller with motor characteristics - 1DoF (no account for ua,up)/1 -> Mux1/1
  3. propeller with motor characteristics - 1DoF (no account for ua,up)1/1 -> Mux1/2
  3. propeller with motor characteristics - 1DoF (no account for ua,up)2/1 -> Mux1/3
  3. propeller with motor characteristics - 1DoF (no account for ua,up)3/1 -> Mux1/4
  Mux1/1 -> output force/1
  input velocity/1 -> Demux/1
  Demux/1 -> 3. propeller with motor characteristics - 1DoF (no account for ua,up)/1
  Demux/2 -> 3. propeller with motor characteristics - 1DoF (no account for ua,up)1/1
  Demux/3 -> 3. propeller with motor characteristics - 1DoF (no account for ua,up)2/1
  Demux/4 -> 3. propeller with motor characteristics - 1DoF (no account for ua,up)3/1

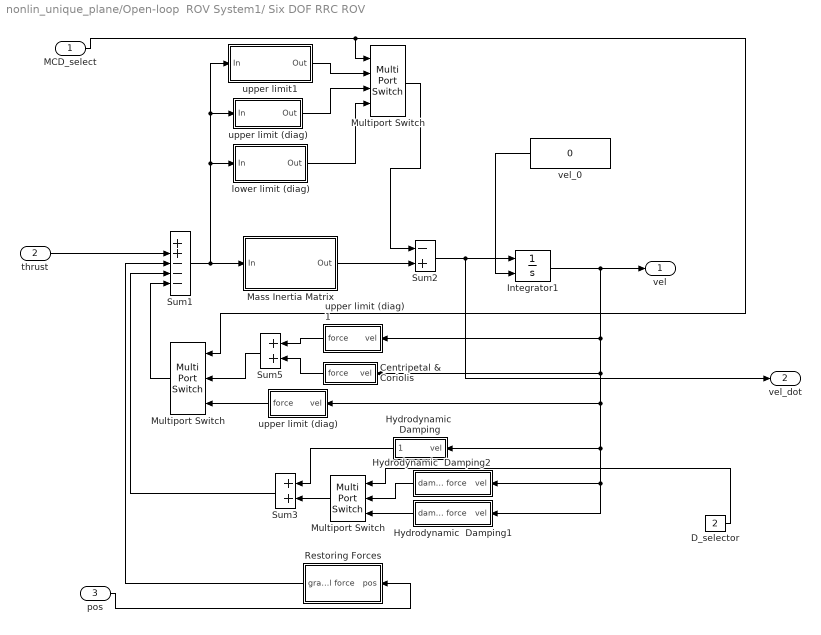
== system nonlin_unique_plane/Open-loop  ROV System1/ Six DOF RRC ROV    ==
  MCD_select : Inport  Port=1  LatchInput=off
  "thrust " : Inport  Port=2  LatchInput=off
  "pos " : Inport  Port=3  LatchInput=off
  Centripetal & Coriolis : Subsystem  Orientation=left  AncestorBlock=rov_design_analysis/ROV Models/1. Six DOF RRC ROV II/Centripetal & Coriolis
      mask Display: disp('C')
  D_selector : Constant  Value=2
  Hydrodynamic  Damping : Subsystem  Orientation=left
      mask Display: disp('D')
  Hydrodynamic  Damping1 : Subsystem  Orientation=left
      mask Display: disp('perturb \nDamping')
  Hydrodynamic  Damping2 : Subsystem  Orientation=left
      mask Display: disp('Zero Perturb')
  Integrator1 : Integrator  InitialConditionSource=external
  Mass Inertia Matrix : Subsystem
      mask Display: disp('inv(MRB+MA)')
  Multiport Switch : MultiPortSwitch  Inputs=3
  "Multiport Switch  " : MultiPortSwitch  Orientation=left  Inputs=2
  "Multiport Switch    " : MultiPortSwitch  Orientation=left  Inputs=2
  Restoring Forces : Subsystem  Orientation=left
      mask Display: disp('Restoring\nForce')
  Sum1 : Sum  Inputs=++---  SaturateOnIntegerOverflow=on  InputSameDT=on
  Sum2 : Sum  Inputs=-+  SaturateOnIntegerOverflow=on  InputSameDT=on
  Sum3 : Sum  Orientation=left  SaturateOnIntegerOverflow=on  InputSameDT=on
  Sum5 : Sum  Orientation=left  SaturateOnIntegerOverflow=on  InputSameDT=on
  lower limit (diag) : Subsystem
      mask Display: disp('Perturb MA')
  upper limit (diag) : Subsystem
      mask Display: disp('Perturb MA')
  "upper limit (diag)   " : Subsystem  Orientation=left
      mask Display: disp('Perturb CA')
  upper limit (diag)   1 : Subsystem  Orientation=left
      mask Display: disp('CA')
  upper limit1 : Subsystem
      mask Display: disp('Zero Perturb')
  vel_0 : Constant  Orientation=left  Value=0  OutDataTypeMode=double
  vel : Outport
  vel_dot : Outport  Port=2
  wires:
  Restoring Forces/1(gravitational force) -> Sum1/3
  "thrust "/1 -> Sum1/2
  Sum1/1 -> Mass Inertia Matrix/1(In), upper limit1/1(In), upper limit (diag)/1(In), lower limit (diag)/1(In)
  "Multiport Switch  "/1 -> Sum1/5
  "pos "/1 -> Restoring Forces/1(pos)
  Mass Inertia Matrix/1(Out) -> Sum2/2
  upper limit1/1(Out) -> Multiport Switch/2
  upper limit (diag)/1(Out) -> Multiport Switch/3
  lower limit (diag)/1(Out) -> Multiport Switch/4
  Multiport Switch/1 -> Sum2/1
  "upper limit (diag)   "/1(force) -> "Multiport Switch  "/3
  Sum5/1 -> "Multiport Switch  "/2
  Hydrodynamic  Damping1/1(damping force) -> "Multiport Switch    "/3
  Hydrodynamic  Damping2/1(damping force) -> "Multiport Switch    "/2
  Sum3/1 -> Sum1/4
  "Multiport Switch    "/1 -> Sum3/2
  Hydrodynamic  Damping/1(damping force) -> Sum3/1
  MCD_select/1 -> Multiport Switch/1, "Multiport Switch  "/1
  upper limit (diag)   1/1(force) -> Sum5/1
  Centripetal & Coriolis/1(force) -> Sum5/2
  Sum2/1 -> Integrator1/1, vel_dot/1
  Integrator1/1 -> vel/1, upper limit (diag)   1/1(vel), Centripetal & Coriolis/1(vel), Hydrodynamic  Damping/1(vel), Hydrodynamic  Damping1/1(vel), Hydrodynamic  Damping2/1(vel), "upper limit (diag)   "/1(vel)
  vel_0/1 -> Integrator1/2
  D_selector/1 -> "Multiport Switch    "/1

== system nonlin_unique_plane/Open-loop  ROV System1/Body Velocity Scope  1 ==
  In : Inport  Port=1  LatchInput=off
  Demux : Demux  Outputs=6
  p : Scope
      settings: TickLabels=on  YMin=-0.125  YMax=0.2  DataFormat=Array
  q : Scope
      settings: TickLabels=on  TimeRange=200  YMin=-0.05  YMax=0.15  DataFormat=Array
  r : Scope
      settings: TickLabels=on  TimeRange=200  YMin=-0.05  YMax=0.15  DataFormat=Array
  u : Scope
      settings: TickLabels=on  TimeRange=50  YMin=-0.025  YMax=0.375  DataFormat=Array
  v : Scope
      settings: TickLabels=on  YMin=-0.02  YMax=0.1  DataFormat=Array
  w : Scope
      settings: TickLabels=on  TimeRange=50  YMin=-0.0025  YMax=0.0375  DataFormat=Array
  wires:
  Demux/1 -> u/1
  Demux/2 -> v/1
  Demux/4 -> p/1
  Demux/3 -> w/1
  In/1 -> Demux/1
  Demux/5 -> q/1
  Demux/6 -> r/1

== system nonlin_unique_plane/Open-loop  ROV System1/Euler Transformation   ==
  vel : Inport  Port=1  LatchInput=off
  Demux : Demux  Outputs=2
  Demux1 : Demux  Outputs=2
  Intregrator2 : Integrator
  Mux1 : Mux  Inputs=2
  Terminator : Terminator
  Transformation matrix R : Subsystem
      mask Display: disp('Transformation R')
  Transformation matrix T : Subsystem
      mask Display: disp('Transformation T')
  eout : Outport  InitialOutput=0
  eout_dot : Outport  Port=2  InitialOutput=0
  wires:
  Mux1/1 -> eout_dot/1, Intregrator2/1
  Intregrator2/1 -> Demux1/1, eout/1
  Demux/2 -> Transformation matrix R/1(angular body  velocity)
  Demux/1 -> Transformation matrix T/1(translational body velocity)
  vel/1 -> Demux/1
  Demux1/2 -> Transformation matrix T/2(angular position), Transformation matrix R/2(angular position)
  Transformation matrix R/1(angular earth velocity) -> Mux1/2
  Transformation matrix T/1(translational earth velocity) -> Mux1/1
  Demux1/1 -> Terminator/1

== system nonlin_unique_plane/Open-loop  ROV System1/Thruster configuration5 ==
  input velocity : Inport  Orientation=up  Port=1  LatchInput=off
  Thruster Matrix : Gain  Gain=T  Multiplication=Matrix(K*u)  SaturateOnIntegerOverflow=on
  output force : Outport  InitialOutput=0
  wires:
  input velocity/1 -> Thruster Matrix/1
  Thruster Matrix/1 -> output force/1

== system nonlin_unique_plane/Open-loop  ROV System1/Thruster configuration8 ==
  input velocity : Inport  Orientation=up  Port=1  LatchInput=off
  3. propeller with motor characteristics - 1DoF (no account for ua,up){,1..3} (4 alike) : rov_design_analysis/Propeller Models/3. propeller with motor characteristics - 1DoF (no account for ua,up)
  Demux : Demux
  Mux1 : Mux
  output force : Outport  InitialOutput=0
  wires:
  3. propeller with motor characteristics - 1DoF (no account for ua,up)/1 -> Mux1/1
  3. propeller with motor characteristics - 1DoF (no account for ua,up)1/1 -> Mux1/2
  3. propeller with motor characteristics - 1DoF (no account for ua,up)2/1 -> Mux1/3
  3. propeller with motor characteristics - 1DoF (no account for ua,up)3/1 -> Mux1/4
  Mux1/1 -> output force/1
  input velocity/1 -> Demux/1
  Demux/1 -> 3. propeller with motor characteristics - 1DoF (no account for ua,up)/1
  Demux/2 -> 3. propeller with motor characteristics - 1DoF (no account for ua,up)1/1
  Demux/3 -> 3. propeller with motor characteristics - 1DoF (no account for ua,up)2/1
  Demux/4 -> 3. propeller with motor characteristics - 1DoF (no account for ua,up)3/1

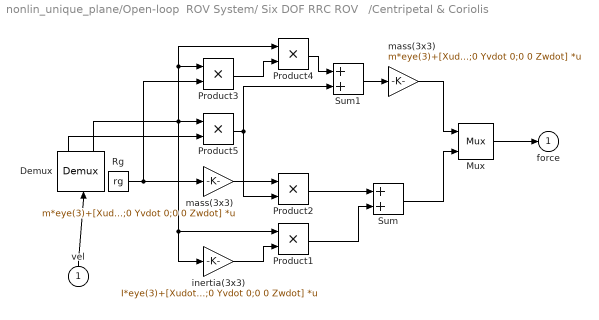
== system nonlin_unique_plane/Open-loop  ROV System/ Six DOF RRC ROV   /Centripetal & Coriolis ==
  vel : Inport  Orientation=up  Port=1  LatchInput=off
  Demux : Demux  Orientation=up  Outputs=2
  Mux : Mux  Inputs=2
  Product{1..5} (5 alike) : Product  SaturateOnIntegerOverflow=on  RndMeth=Zero  InputSameDT=on
  Rg : Constant  Value=rg
  Sum : Sum  SaturateOnIntegerOverflow=on  InputSameDT=on
  Sum1 : Sum  SaturateOnIntegerOverflow=on  InputSameDT=on
  inertia(3x3) : Gain  Gain=I*eye(3)+[Xudot 0 0;0 Yvdot 0;0 0 Zwdot]  Multiplication=Matrix(K*u)  SaturateOnIntegerOverflow=on
  "mass(3x3) " : Gain  Gain=m*eye(3)+[Xudot 0 0;0 Yvdot 0;0 0 Zwdot]  Multiplication=Matrix(K*u)  SaturateOnIntegerOverflow=on
  "mass(3x3)   " : Gain  Gain=m*eye(3)+[Xudot 0 0;0 Yvdot 0;0 0 Zwdot]  Multiplication=Matrix(K*u)  SaturateOnIntegerOverflow=on
  force : Outport  InitialOutput=0
  wires:
  Product1/1 -> Sum/2
  "mass(3x3)   "/1 -> Product2/1
  Product2/1 -> Sum/1
  Rg/1 -> Product3/2, "mass(3x3)   "/1
  Product3/1 -> Product4/2
  Product4/1 -> Sum1/1
  Product5/1 -> Product2/2, Sum1/2
  Sum1/1 -> "mass(3x3) "/1
  Demux/2 -> Product5/1, Product3/1, Product4/1, Product1/1, inertia(3x3)/1
  Demux/1 -> Product5/2
  vel/1 -> Demux/1
  inertia(3x3)/1 -> Product1/2
  "mass(3x3) "/1 -> Mux/1
  Sum/1 -> Mux/2
  Mux/1 -> force/1

== system nonlin_unique_plane/Open-loop  ROV System/ Six DOF RRC ROV   /Hydrodynamic  Damping ==
  vel : Inport  Port=1  LatchInput=off
  D linear : Gain  Gain=-diag(DQL)  SaturateOnIntegerOverflow=on
  damping force : Outport  InitialOutput=0
  wires:
  vel/1 -> D linear/1
  D linear/1 -> damping force/1

== system nonlin_unique_plane/Open-loop  ROV System/ Six DOF RRC ROV   /Hydrodynamic  Damping1 ==
  vel : Inport  Port=1  LatchInput=off
  D quadratic : Gain  Gain=-diag(DQ)  SaturateOnIntegerOverflow=on
  Product : Product  SaturateOnIntegerOverflow=on  RndMeth=Zero  InputSameDT=on
  |u| : Abs  SaturateOnIntegerOverflow=on
  damping force : Outport  InitialOutput=0
  wires:
  Product/1 -> D quadratic/1
  vel/1 -> Product/1, |u|/1
  |u|/1 -> Product/2
  D quadratic/1 -> damping force/1

== system nonlin_unique_plane/Open-loop  ROV System/ Six DOF RRC ROV   /Hydrodynamic  Damping2 ==
  vel : Inport  Port=1  LatchInput=off
  D quadratic : Gain  Gain=0  SaturateOnIntegerOverflow=on
  damping force : Outport  InitialOutput=0
  wires:
  D quadratic/1 -> damping force/1
  vel/1 -> D quadratic/1

== system nonlin_unique_plane/Open-loop  ROV System/ Six DOF RRC ROV   /Mass Inertia Matrix ==
  In : Inport  Port=1  LatchInput=off
  inverse M : Gain  Gain=inv(M-Ma)  Multiplication=Matrix(K*u)  SaturateOnIntegerOverflow=on
  Out : Outport
  wires:
  inverse M/1 -> Out/1
  In/1 -> inverse M/1

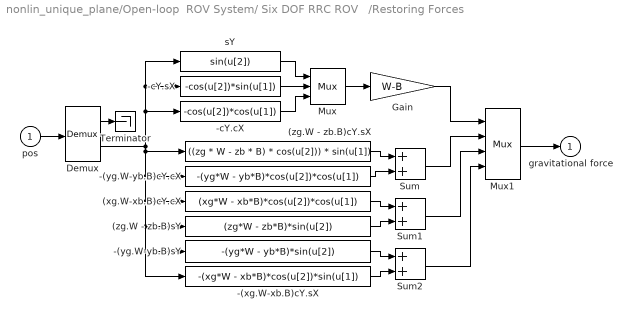
== system nonlin_unique_plane/Open-loop  ROV System/ Six DOF RRC ROV   /Restoring Forces ==
  pos : Inport  Port=1  LatchInput=off
  (xg.W-xb.B)cY.cX : Fcn  Expr=(xg*W - xb*B)*cos(u[2])*cos(u[1])
  (zg.W - zb.B)cY.sX : Fcn  Expr=((zg * W - zb * B) * cos(u[2])) * sin(u[1])
  (zg.W - zb.B)sY : Fcn  Expr=(zg*W - zb*B)*sin(u[2])
  -(xg.W-xb.B)cY.sX : Fcn  Expr=-(xg*W - xb*B)*cos(u[2])*sin(u[1])
  -(yg.W-yb.B)cY.cX : Fcn  Expr=-(yg*W - yb*B)*cos(u[2])*cos(u[1])
  -(yg.W-yb.B)sY : Fcn  Expr=-(yg*W - yb*B)*sin(u[2])
  -cY.cX : Fcn  Expr=-cos(u[2])*cos(u[1])
  -cY.sX : Fcn  Expr=-cos(u[2])*sin(u[1])
  Demux : Demux  Outputs=2
  Gain : Gain  Gain=W-B  SaturateOnIntegerOverflow=on
  Mux : Mux  Inputs=3
  Mux1 : Mux
  Sum : Sum  SaturateOnIntegerOverflow=on  InputSameDT=on
  Sum1 : Sum  SaturateOnIntegerOverflow=on  InputSameDT=on
  Sum2 : Sum  SaturateOnIntegerOverflow=on  InputSameDT=on
  Terminator : Terminator
  sY : Fcn  Expr=sin(u[2])
  gravitational force : Outport  InitialOutput=0
  wires:
  Sum2/1 -> Mux1/4
  -(yg.W-yb.B)sY/1 -> Sum2/1
  -(xg.W-xb.B)cY.sX/1 -> Sum2/2
  Sum1/1 -> Mux1/3
  (xg.W-xb.B)cY.cX/1 -> Sum1/1
  (zg.W - zb.B)sY/1 -> Sum1/2
  Sum/1 -> Mux1/2
  (zg.W - zb.B)cY.sX/1 -> Sum/1
  -(yg.W-yb.B)cY.cX/1 -> Sum/2
  Gain/1 -> Mux1/1
  Mux/1 -> Gain/1
  -cY.cX/1 -> Mux/3
  -cY.sX/1 -> Mux/2
  sY/1 -> Mux/1
  Mux1/1 -> gravitational force/1
  Demux/2 -> -(xg.W-xb.B)cY.sX/1, -(yg.W-yb.B)sY/1, (zg.W - zb.B)sY/1, (xg.W-xb.B)cY.cX/1, -(yg.W-yb.B)cY.cX/1, (zg.W - zb.B)cY.sX/1, sY/1, -cY.sX/1, -cY.cX/1
  Demux/1 -> Terminator/1
  pos/1 -> Demux/1

== system nonlin_unique_plane/Open-loop  ROV System/ Six DOF RRC ROV   /lower limit (diag) ==
  In : Inport  Port=1  LatchInput=off
  inverse M : Gain  Gain=-diag([21.1403-21.0981 51.7012-51.0026 92.451-91.837 3.6191-3.576 2.6427-2.7687 2.3033-2.3493])  Multiplication=Matrix(K*u)  SaturateOnIntegerOverflow=on
  Out : Outport
  wires:
  inverse M/1 -> Out/1
  In/1 -> inverse M/1

== system nonlin_unique_plane/Open-loop  ROV System/ Six DOF RRC ROV   /upper limit (diag) ==
  In : Inport  Port=1  LatchInput=off
  inverse M : Gain  Gain=-diag([21.724-21.1403 51.7013-51.7012 94.3-92.451 4.2176-3.6191 7.1148-2.6427 4.7673-2.3033])  Multiplication=Matrix(K*u)  SaturateOnIntegerOverflow=on
  Out : Outport
  wires:
  inverse M/1 -> Out/1
  In/1 -> inverse M/1

== system nonlin_unique_plane/Open-loop  ROV System/ Six DOF RRC ROV   /upper limit (diag)    ==
  note: 7 8 9 10 11 12
  note: 1 2 3 4 5 6
  vel : Inport  Port=1  LatchInput=off
  (zg.W - zb.B)cY.sX : Fcn  Expr=-u[9]*u[3]*u[5]+u[8]*u[2]*u[6]
  (zg.W - zb.B)cY.sX1 : Fcn  Expr=u[9]*u[3]*u[4]-u[7]*u[1]*u[6]
  (zg.W - zb.B)cY.sX2 : Fcn  Expr=-u[8]*u[2]*u[4]+u[7]*u[1]*u[5]
  (zg.W - zb.B)cY.sX3 : Fcn  Expr=-u[9]*u[3]*u[2]+u[8]*u[2]*u[3]-u[12]*u[6]*u[5]+u[11]*u[5]*u[6]
  (zg.W - zb.B)cY.sX4 : Fcn  Expr=u[9]*u[3]*u[1]-u[7]*u[1]*u[3]+u[6]*u[12]*u[4]-u[4]*u[10]*u[6]
  (zg.W - zb.B)cY.sX5 : Fcn  Expr=-u[8]*u[2]*u[1]+u[7]*u[1]*u[2]-u[11]*u[5]*u[4]+u[10]*u[4]*u[5]
  Mux1 : Mux  Inputs=6
  Mux3 : Mux  Inputs=2
  Rg1 : Constant  Value="[MaU(1)  MaU(2)  MaU(3)  MaU(4)  MaU(5)  MaU(6) ]'"
  force : Outport
  wires:
  Mux1/1 -> force/1
  (zg.W - zb.B)cY.sX/1 -> Mux1/1
  (zg.W - zb.B)cY.sX1/1 -> Mux1/2
  (zg.W - zb.B)cY.sX2/1 -> Mux1/3
  (zg.W - zb.B)cY.sX3/1 -> Mux1/4
  (zg.W - zb.B)cY.sX4/1 -> Mux1/5
  (zg.W - zb.B)cY.sX5/1 -> Mux1/6
  vel/1 -> Mux3/1
  Rg1/1 -> Mux3/2
  Mux3/1 -> (zg.W - zb.B)cY.sX/1, (zg.W - zb.B)cY.sX1/1, (zg.W - zb.B)cY.sX4/1, (zg.W - zb.B)cY.sX5/1, (zg.W - zb.B)cY.sX3/1, (zg.W - zb.B)cY.sX2/1

== system nonlin_unique_plane/Open-loop  ROV System/ Six DOF RRC ROV   /upper limit (diag)   1 ==
  note: 7 8 9 10 11 12
  note: 1 2 3 4 5 6
  vel : Inport  Port=1  LatchInput=off
  (zg.W - zb.B)cY.sX : Fcn  Expr=-u[9]*u[3]*u[5]+u[8]*u[2]*u[6]
  (zg.W - zb.B)cY.sX1 : Fcn  Expr=u[9]*u[3]*u[4]-u[7]*u[1]*u[6]
  (zg.W - zb.B)cY.sX2 : Fcn  Expr=-u[8]*u[2]*u[4]+u[7]*u[1]*u[5]
  (zg.W - zb.B)cY.sX3 : Fcn  Expr=-u[9]*u[3]*u[2]+u[8]*u[2]*u[3]-u[12]*u[6]*u[5]+u[11]*u[5]*u[6]
  (zg.W - zb.B)cY.sX4 : Fcn  Expr=u[9]*u[3]*u[1]-u[7]*u[1]*u[3]+u[6]*u[12]*u[4]-u[4]*u[10]*u[6]
  (zg.W - zb.B)cY.sX5 : Fcn  Expr=-u[8]*u[2]*u[1]+u[7]*u[1]*u[2]-u[11]*u[5]*u[4]+u[10]*u[4]*u[5]
  Mux1 : Mux  Inputs=6
  Mux3 : Mux  Inputs=2
  Rg1 : Constant  Value="[Ma(1)  Ma(2)  Ma(3)  Ma(4)  Ma(5)  Ma(6) ]'"
  force : Outport
  wires:
  Mux1/1 -> force/1
  (zg.W - zb.B)cY.sX/1 -> Mux1/1
  (zg.W - zb.B)cY.sX1/1 -> Mux1/2
  (zg.W - zb.B)cY.sX2/1 -> Mux1/3
  (zg.W - zb.B)cY.sX3/1 -> Mux1/4
  (zg.W - zb.B)cY.sX4/1 -> Mux1/5
  (zg.W - zb.B)cY.sX5/1 -> Mux1/6
  vel/1 -> Mux3/1
  Rg1/1 -> Mux3/2
  Mux3/1 -> (zg.W - zb.B)cY.sX/1, (zg.W - zb.B)cY.sX1/1, (zg.W - zb.B)cY.sX4/1, (zg.W - zb.B)cY.sX5/1, (zg.W - zb.B)cY.sX3/1, (zg.W - zb.B)cY.sX2/1

== system nonlin_unique_plane/Open-loop  ROV System/ Six DOF RRC ROV   /upper limit1 ==
  In : Inport  Port=1  LatchInput=off
  inverse M : Gain  Gain=0  Multiplication=Matrix(K*u)  SaturateOnIntegerOverflow=on
  Out : Outport
  wires:
  inverse M/1 -> Out/1
  In/1 -> inverse M/1
